simulink model "PBVS"  (R2020b)
settings: Solver=VariableStepAuto  StartTime=0.0  StopTime=10  RelTol=1e-3
values from neighbouring files (symbols this model uses):
  dT = 1/frequency    (= 0.005)    [init_PBVS.m]
  f = 0.5    [init_PBVS.m]
  init_pose = [C ; ang']    [init_PBVS.m]
  Kp = 1*eye(6)    [init_PBVS.m]
  O = [0; 0; 0]    [init_PBVS.m]
  p1 = [1.7; 0.65; 0.6]    [init_PBVS.m]
  ref = [-0.2; 0; 0; pi/2; 0 ; pi/2]    [init_PBVS.m]
libraries: simulink x1
settings Model: Creator=Acer  LastModifiedBy=antonio

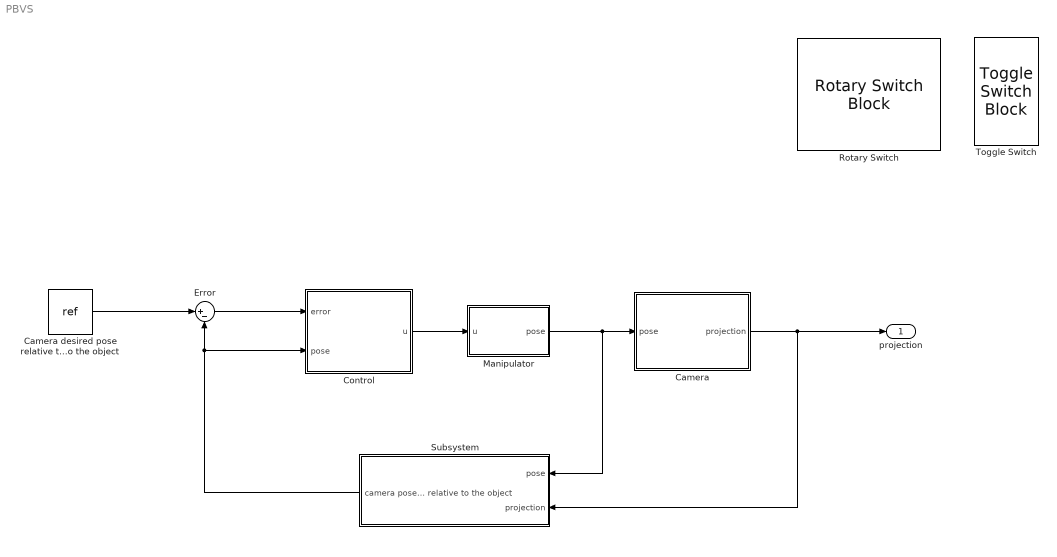
== system PBVS ==
  Camera : Subsystem
  Camera desired pose relative to the object : Constant  Value=ref  SampleTime=-1
  Control : Subsystem
  Error : Sum  Inputs=|+-
  Manipulator : Subsystem
  Rotary Switch : RotarySwitchBlock  LabelPosition=Bottom
      settings: Values={{'Off', 'Low', 'Medium', 'High'}, [0 0.1 0.2 0.3]}
  Subsystem : Subsystem
  Toggle Switch : ToggleSwitchBlock  LabelPosition=Bottom
      settings: Values={{'Off', 'On'}, [0 1]}
  projection : Outport
  wires:
  Camera/1(projection) -> Subsystem/2(projection), projection/1
  Control/1(u) -> Manipulator/1(u)
  Error/1 -> Control/1(error)
  Manipulator/1(pose) -> Subsystem/1(pose), Camera/1(pose)
  Camera desired pose relative to the object/1 -> Error/1
  Subsystem/1(camera pose relative to the object) -> Control/2(pose), Error/2

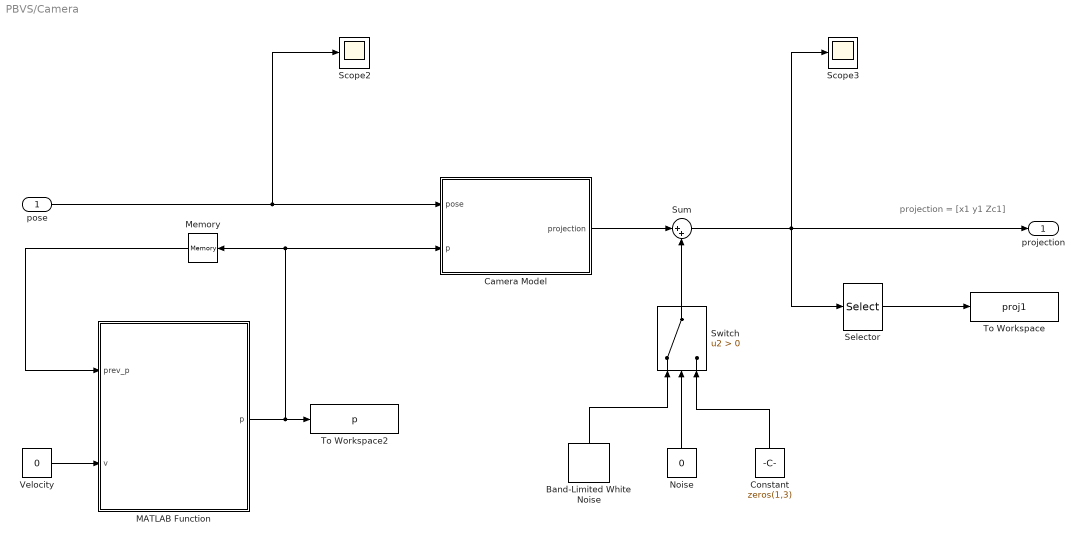
== system PBVS/Camera ==
  note: projection = [x1 y1 Zc1]
  pose : Inport
  Band-Limited White Noise : simulink/Sources/Band-Limited White Noise  Cov=[0.00001 0.00001 0.00001]  Ts=0.01  seed=[23341 10 14]
  Camera Model : MATLAB Function  TreatAsAtomicUnit=on
  Constant : Constant  Value=zeros(1,3)
  MATLAB Function : MATLAB Function  TreatAsAtomicUnit=on  SystemSampleTime=dT
  Memory : Memory  InitialCondition=[p1]
  Noise : Constant  Value=0
  Scope2 : Scope
  Scope3 : Scope
  Selector : Selector  InputPortWidth=3  IndexOptions=Index vector (dialog)  Indices=[1 2]  OutputSizes=1
  Sum : Sum  Inputs=|++
  Switch : Switch  Criteria=u2 > Threshold
  To Workspace : ToWorkspace  VariableName=proj1  SampleTime=0.1
  To Workspace2 : ToWorkspace  VariableName=p  SampleTime=0.1
  Velocity : Constant  Value=0  SampleTime=dT
  projection : Outport
  wires:
  pose/1 -> Scope2/1, Camera Model/1(pose)
  Selector/1 -> To Workspace/1
  Camera Model/1(projection) -> Sum/1
  Sum/1 -> Scope3/1, Selector/1, projection/1
  Switch/1 -> Sum/2
  Noise/1 -> Switch/2
  Band-Limited White Noise/1 -> Switch/1
  Constant/1 -> Switch/3
  MATLAB Function/1(p) -> To Workspace2/1, Camera Model/2(p), Memory/1
  Memory/1 -> MATLAB Function/1(prev_p)
  Velocity/1 -> MATLAB Function/2(v)

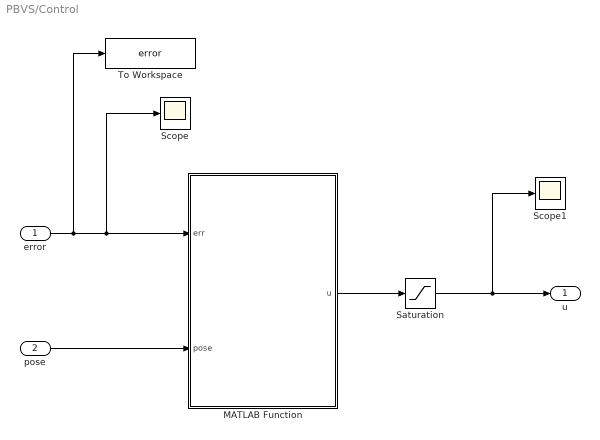
== system PBVS/Control ==
  error : Inport
  pose : Inport  Port=2
  MATLAB Function : MATLAB Function  TreatAsAtomicUnit=on  SystemSampleTime=1/200
  Saturation : Saturate
  Scope : Scope
  Scope1 : Scope
  To Workspace : ToWorkspace  VariableName=error  SampleTime=0.1
  u : Outport
  wires:
  error/1 -> To Workspace/1, Scope/1, MATLAB Function/1(err)
  pose/1 -> MATLAB Function/2(pose)
  MATLAB Function/1(u) -> Saturation/1
  Saturation/1 -> u/1, Scope1/1

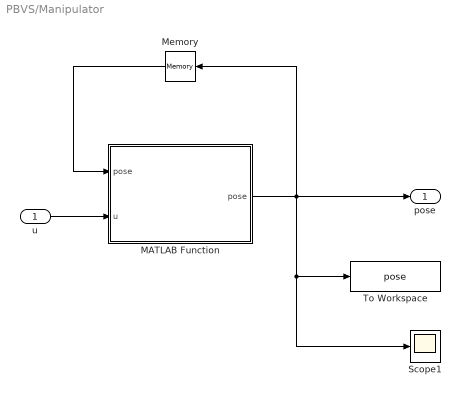
== system PBVS/Manipulator ==
  u : Inport
  MATLAB Function : MATLAB Function  TreatAsAtomicUnit=on  SystemSampleTime=1/200
  Memory : Memory  InitialCondition=init_pose
  Scope1 : Scope
  To Workspace : ToWorkspace  VariableName=pose  SampleTime=0.1
  pose : Outport
  wires:
  u/1 -> MATLAB Function/2(u)
  Memory/1 -> MATLAB Function/1("pose ")
  MATLAB Function/1(pose) -> pose/1, Memory/1, Scope1/1, To Workspace/1

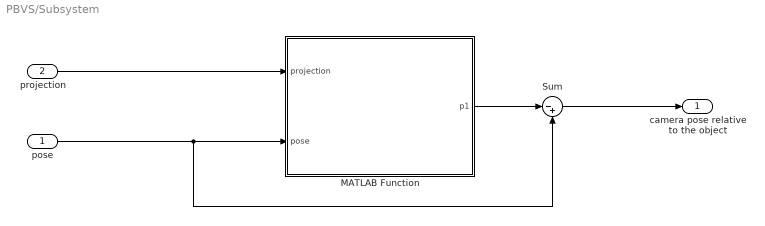
== system PBVS/Subsystem ==
  pose : Inport
  projection : Inport  Port=2
  MATLAB Function : MATLAB Function  TreatAsAtomicUnit=on
  Sum : Sum  Inputs=|-+
  camera pose relative to the object : Outport
  wires:
  MATLAB Function/1(p1) -> Sum/1
  Sum/1 -> camera pose relative to the object/1
  pose/1 -> Sum/2, MATLAB Function/2(pose)
  projection/1 -> MATLAB Function/1(projection)

== matlab function PBVS/Control/MATLAB Function ==
  data: err input; pose input; Kp parameter; u output; ref parameter
function u = fcn(err, pose, Kp, ref)

% pose : relative pose between camera and object
% ref : desired relative pose between camera and object
% err : error between desired and actual pose of the camera relative to the object

ang = zeros(3, 1);
ang(1) = pose(4) - ref(4);  % camera's orientation 
ang(2) = pose(5) - ref(5);
ang(3) = pose(6) - ref(6);

% Trasformation
Rx = [1   0       0   ;
      0 cos(ang(1)) -sin(ang(1));
      0 sin(ang(1)) cos(ang(1))];

Ry = [cos(ang(2)) 0 sin(ang(2)) ;
       0     1   0    ;
     -sin(ang(2)) 0 cos(ang(2))];
 
Rz = [cos(ang(3)) -sin(ang(3)) 0;
      sin(ang(3))  cos(ang(3)) 0;
       0      0     1];

Rd = Rz * Ry * Rx; % rotation matrix 

J2 = [1     sin(ang(1))*tan(ang(2))    cos(ang(1))*tan(ang(2));
      0           cos(ang(1))                  -sin(ang(1));
      0     sin(ang(1))/cos(ang(2))    cos(ang(1))/cos(ang(2)) ];

J = eye(6);  % Jacobian J(q)

Ja = [Rd' zeros(3); zeros(3) J2^-1] * J;

% PBVS control Law
u = Ja^-1 * (Kp * err);

== matlab function PBVS/Camera/Camera Model ==
  data: projection output; f parameter; O parameter; pose input; p input
function projection = proj(f, O, pose, p)
% function that computes the projection of the point in the image plane
% f : focal lenght
% O : world origin frame
% pose: pose of the camera
% p : point position

d = pose(1:3) - O;    % camera's position in world frame
ang = pose(4:6);      % camera's orientation 
p1 = p;               


%%
Rx = [1   0       0   ;
      0 cos(ang(1)) -sin(ang(1));
      0 sin(ang(1)) cos(ang(1))];

Ry = [cos(ang(2)) 0 sin(ang(2)) ;
       0     1   0    ;
     -sin(ang(2)) 0 cos(ang(2))];
 
Rz = [cos(ang(3)) -sin(ang(3)) 0;
      sin(ang(3))  cos(ang(3)) 0;
       0      0     1];


Rc = Rz * Ry * Rx;


Twc = [Rc            d;
      zeros(1,3)     1];

%%
P = diag([f,f,1]) * [eye(3), zeros(3,1)]; % camera projection matrix

p_cam1 = Twc^-1 * [p1; 1];   % point position in camera frame

p_tilde1 = P * p_cam1;

x_proj1 = p_tilde1(1)/p_cam1(3);
y_proj1 = p_tilde1(2)/p_cam1(3);
Zc1 = p_cam1(3);


projection  = [x_proj1; y_proj1; Zc1]; %; x_proj2; y_proj2; Zc2];
% x_proj1, y_proj1 : point projection in image plane
% Zc1 : point depth in camera frame

end

== matlab function PBVS/Manipulator/MATLAB Function ==
  data: pose input; u input; pose output; dT parameter
function pose = fcn(pose, u, dT)

position = zeros(3, 1);
angle = zeros(3, 1);
ang = u(4:6);

Rx = [1   0       0   ;
      0 cos(ang(1)) -sin(ang(1));
      0 sin(ang(1)) cos(ang(1))];

Ry = [cos(ang(2)) 0 sin(ang(2)) ;
       0     1   0    ;
     -sin(ang(2)) 0 cos(ang(2))];
 
Rz = [cos(ang(3)) -sin(ang(3)) 0;
      sin(ang(3))  cos(ang(3)) 0;
       0      0     1];

J1 = Rz * Ry * Rx;

J2 = [1     sin(ang(1))*tan(ang(2))    cos(ang(1))*tan(ang(2));
      0           cos(ang(1))                  -sin(ang(1));
      0     sin(ang(1))/cos(ang(2))    cos(ang(1))/cos(ang(2)) ];


position = pose(1:3) + J1 * u(1:3) * dT;
angle = pose(4:6) + J2 * ang * dT;
pose = [position; angle];

== matlab function PBVS/Camera/MATLAB Function ==
  data: prev_p input; p output; v input; dT parameter
function p = fcn(prev_p ,v, dT)

p1 = prev_p;

p1 = p1 + [0; v; 0] * dT;

p = p1;

== matlab function PBVS/Subsystem/MATLAB Function ==
  data: projection input; p1 output; pose input; O parameter; f parameter
function p1  = fcn(projection, pose, O, f)
% function that computes the point position in camera frame from the point
% projection in the image plane 
% pose : pose of the camera 

x1 = projection(1); % x projection in the image plane
y1 = projection(2); % y projection in the image plane 
Zc1 = projection(3); % point depth in camera frame 

d = pose(1:3) - O;    % camera's position in world frame
ang = pose(4:6);      % camera's orientation 

%%
Rx = [1   0       0   ;
      0 cos(ang(1)) -sin(ang(1));
      0 sin(ang(1)) cos(ang(1))];

Ry = [cos(ang(2)) 0 sin(ang(2)) ;
       0     1   0    ;
     -sin(ang(2)) 0 cos(ang(2))];
 
Rz = [cos(ang(3)) -sin(ang(3)) 0;
      sin(ang(3))  cos(ang(3)) 0;
       0      0     1];


Rc = Rz * Ry * Rx;


Twc = [Rc            d;
      zeros(1,3)     1];

P = diag([f,f,1]) * [eye(3), zeros(3,1)]; % camera projection matrix


p_tilde1 = [x1 * Zc1; y1 * Zc1; Zc1];
p_cam1 = P(:, 1:3)^-1 * p_tilde1;

p1_hom = Twc * [p_cam1; 1];
p1 = [p1_hom(1:3); 0; 0; 0];   % [p1(1) p1(2) p1(3)] : point position in camera frame 
                               % [p1(4) p1(5) p1(6)] : point orientation in world frame 


% p1 = Twc * pinv(P) * [x1*Zc1; y1*Zc1; Zc1];
% p2 = Twc * pinv(P) * [x2*Zc2; y2*Zc2; Zc2];
